simulink model "BrainBC"  (R2019a)
settings: Solver=VariableStepAuto  StartTime=0.0  StopTime=10.0  RelTol=1e-3
undefined symbols (not defined in the file): GBC_B, Q_gB, T_gB, V_gBC, V_gBF
settings Model: Creator=jcp2  LastModifiedBy=rache

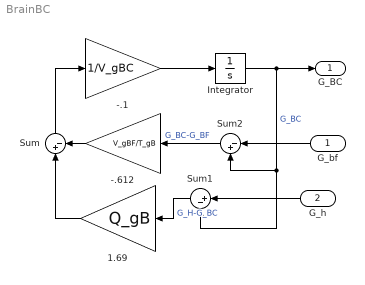
== system BrainBC ==
  G_bf : Inport
  G_h : Inport  Port=2
  -.1 : Gain  Gain=1/V_gBC
  -.612 : Gain  Gain=V_gBF/T_gB
  "1.69 " : Gain  Gain=Q_gB
  Integrator : Integrator  InitialCondition=GBC_B  LimitOutput=on  LowerSaturationLimit=0
  Sum : Sum  Inputs=|+-
  Sum1 : Sum  Inputs=|+-
  Sum2 : Sum  Inputs=|-+
  G_BC : Outport
  wires:
  Integrator/1 -> Sum2/2, Sum1/2, G_BC/1  "G_BC"
  G_h/1 -> Sum1/1
  G_bf/1 -> Sum2/1
  Sum2/1 -> -.612/1  "G_BC-G_BF"
  Sum1/1 -> "1.69 "/1  "G_H-G_BC"
  "1.69 "/1 -> Sum/1
  -.612/1 -> Sum/2
  Sum/1 -> -.1/1
  -.1/1 -> Integrator/1
